simulink model "PID0"  (R2020b)
settings: Solver=VariableStepAuto  StartTime=0.0  StopTime=1  RelTol=1e-3
values from neighbouring files (symbols this model uses):
  Kd = 0.8    [prob4_data.sldd]
  Ki = 40.0    [prob4_data.sldd]
  Kp = 500.0    [prob4_data.sldd]
  n = 119000.0    [prob4_data.sldd]
settings Model: DataDictionary=prob4_data.sldd  Creator=Varun  LastModifiedBy=Varun
settings DataIOCC: SaveOutput=off  SaveTime=off

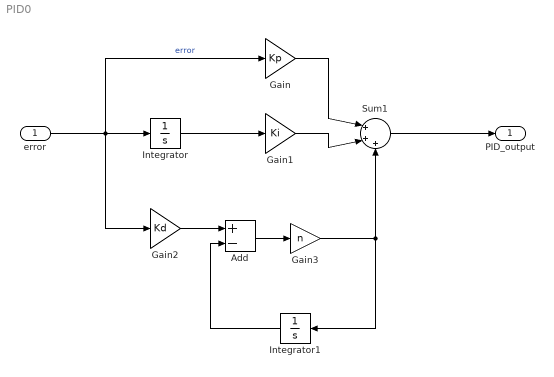
== system PID0 ==
  error : Inport  OutDataTypeStr=double  PortDimensions=1  SampleTime=0
  Add : Sum  Inputs=+-
  Gain : Gain  Gain=Kp
  Gain1 : Gain  Gain=Ki
  Gain2 : Gain  Gain=Kd
  Gain3 : Gain  Gain=n
  Integrator : Integrator
  Integrator1 : Integrator
  Sum1 : Sum  Inputs=|+++
  PID_output : Outport  OutDataTypeStr=double  PortDimensions=1  SampleTime=0
  wires:
  Sum1/1 -> PID_output/1
  error/1 -> Gain2/1, Integrator/1, Gain/1  "error"
  Integrator/1 -> Gain1/1
  Gain1/1 -> Sum1/2
  Gain/1 -> Sum1/1
  Gain2/1 -> Add/1
  Add/1 -> Gain3/1
  Gain3/1 -> Integrator1/1, Sum1/3
  Integrator1/1 -> Add/2
